simulink model "partieDRL"  (R2024a)
settings: Solver=ode45  StartTime=0.0  StopTime=0.04  RelTol=1e-3  EnableMultiTasking=on
libraries: spsDetailedThyristorLib x16, spsVoltageMeasurementLib x5, spsACVoltageSourceLib x4, spsCurrentMeasurementLib x4, spsDCVoltageSourceLib x4, spsSeriesRLCBranchLib x4, spsDiodeLib x1, spspowerguiLib x1, sps_lib x1
settings Model: Creator=ianyl  LastModifiedBy=ianyl
settings SolverCC: AlgebraicLoopSolver=TrustRegion
settings DataIOCC: LimitDataPoints=on  SaveFormat=Array  ReturnWorkspaceOutputs=off
settings OptimizationCC: LifeSpan=inf
settings DebuggingCC: UnconnectedInputMsg=warning  UnconnectedOutputMsg=warning  UnconnectedLineMsg=warning  SFUnexpectedBacktrackingDiag=warning  SFNoUnconditionalDefaultTransitionDiag=warning  SFExecutionAtInitializationDiag=none  ArithmeticOperatorsInVariantConditions=warning
settings HardwareCC: ProdBitPerPointer=32  ProdBitPerSizeT=32  ProdBitPerPtrDiffT=32  ProdLargestAtomicFloat=None  ProdIntDivRoundTo=Undefined  ProdEndianess=Unspecified  ProdWordSize=32  ProdHWDeviceType=32-bit Generic
settings ModelReferenceCC: PropagateSignalLabelsOutOfModel=off
settings SFSimCC: SimUseLocalCustomCode=off  CustomCodeUndefinedFunction=UseInterfaceOnly
settings RTWCC: RTWUseLocalCustomCode=off  GPUComputeCapability=3.5
settings CodeAppCC: StateflowObjectComments=on
settings GRTTargetCC: TargetLangStandard=C89/C90 (ANSI)
settings ConfigComp: CovMetricSettings=dw  CovSaveCumulativeToWorkspaceVar=on  CovSaveSingleToWorkspaceVar=on  CovExternalEMLEnable=off
settings SimscapeCC: SimscapeNormalizeSystem=off

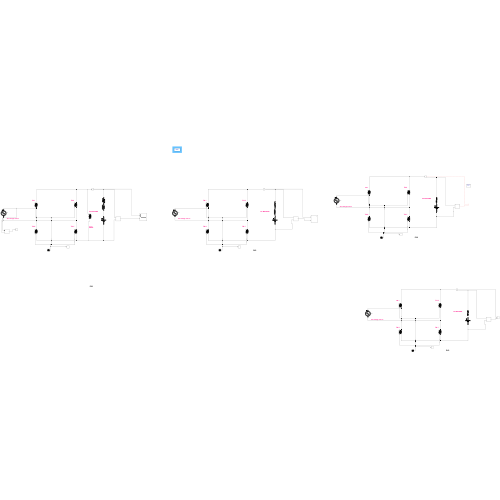
[thumbnail: Simulink's stored preview of the top-level diagram]
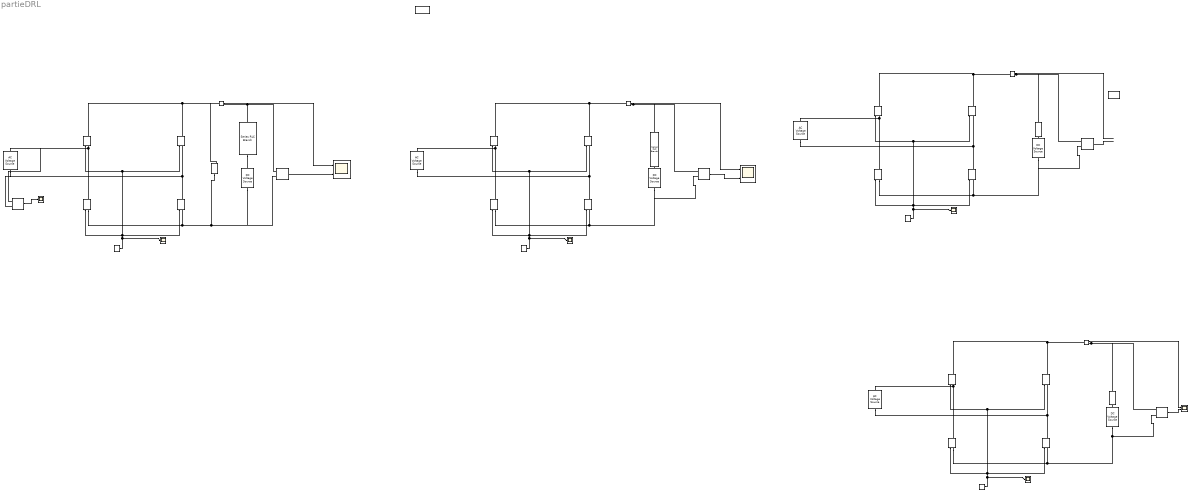
== system partieDRL ==
  note: DRL
  note: PI/3
  note: DC MACHINE
  note: AC voltage source
  note: TH 2'
  note: TH 1'
  note: TH 2
  note: TH 1
  note: PI/2
  note: DC MACHINE
  note: AC voltage source
  note: TH 2'
  note: TH 1'
  note: TH 2
  note: TH 1
  note: PI/2
  note: DC MACHINE
  note: AC voltage source
  note: TH 2'
  note: TH 1'
  note: TH 2
  note: TH 1
  note: PI/2
  note: DC MACHINE
  note: AC voltage source
  note: TH 2'
  note: TH 1'
  note: TH 2
  note: TH 1
  AC : spsACVoltageSourceLib/AC Voltage Source  Amplitude=320.1779  Phase=0  Frequency=50  SampleTime=0  Measurements=None  BusType=swing  Pref=10e3  Qref=0  Qmin=-inf  Qmax=+inf
  AC1 : spsACVoltageSourceLib/AC Voltage Source  Amplitude=320.1779  Phase=0  Frequency=50  SampleTime=0  Measurements=None  BusType=swing  Pref=10e3  Qref=0  Qmin=-inf  Qmax=+inf
  AC2 : spsACVoltageSourceLib/AC Voltage Source  Amplitude=340.4  Phase=0  Frequency=50  SampleTime=0  Measurements=None  BusType=swing  Pref=10e3  Qref=0  Qmin=-inf  Qmax=+inf
  AC3 : spsACVoltageSourceLib/AC Voltage Source  Amplitude=340.4  Phase=0  Frequency=50  SampleTime=0  Measurements=None  BusType=swing  Pref=10e3  Qref=0  Qmin=-inf  Qmax=+inf
  Current Measurement{,1..3} (4 alike) : spsCurrentMeasurementLib/Current Measurement  PhasorSimulation=off  OutputType=Complex  PSBequivalent=0
  DC Voltage Source : spsDCVoltageSourceLib/DC Voltage Source  Amplitude=142.528  Measurements=None
  DC Voltage Source1 : spsDCVoltageSourceLib/DC Voltage Source  Amplitude=92.48  Measurements=None
  DC Voltage Source2 : spsDCVoltageSourceLib/DC Voltage Source  Amplitude=100  Measurements=None
  DC Voltage Source3 : spsDCVoltageSourceLib/DC Voltage Source  Amplitude=100  Measurements=None
  Detailed Thyristor{,1..15} (16 alike) : spsDetailedThyristorLib/Detailed Thyristor  Ron=0.001  Lon=1e-3  Vf=0.8  IL=0.1  Tq=100e-6  IC=0  Rs=500  Cs=250e-9  Measurements=on
      settings: LibrarySourceBlock=sps_lib/Power Electronics/Detailed Thyristor
  Diode : spsDiodeLib/Diode  Ron=0.001  Lon=0  Vf=0.8  IC=0  UseSnubber=off  Rs=500  Cs=250e-9  Measurements=on
  Pulse Generator : DiscretePulseGenerator  PulseType=Time based  Amplitude=5  Period=0.01  PulseWidth=30  PhaseDelay=3.333333*10^(-3)
  Pulse Generator2 : DiscretePulseGenerator  PulseType=Time based  Amplitude=5  Period=0.01  PulseWidth=30  PhaseDelay=5*10^(-3)
  Pulse Generator3 : DiscretePulseGenerator  PulseType=Time based  Amplitude=5  Period=0.01  PulseWidth=30  PhaseDelay=5*10^(-3)
  Pulse Generator4 : DiscretePulseGenerator  PulseType=Time based  Amplitude=5  Period=0.01  PulseWidth=30  PhaseDelay=5*10^(-3)
  Scope : Scope  NumInputPorts=2
  Scope{1..2,4..6} (5 alike) : Scope
  Scope3 : Scope  NumInputPorts=2
  Scope7 : Scope  NumInputPorts=2
  Series RLC Branch : spsSeriesRLCBranchLib/Series RLC Branch  LConnTagsString=__new0  RConnTagsString=__new0  BranchType=RL  Resistance=2.33  Inductance=0.055  SetiL0=off  InitialCurrent=0  Capacitance=1e-6  Setx0=off  InitialVoltage=0  Measurements=None
  Series RLC Branch1 : spsSeriesRLCBranchLib/Series RLC Branch  LConnTagsString=__new0  RConnTagsString=__new0  BranchType=RL  Resistance=2.33  Inductance=0.286  SetiL0=off  InitialCurrent=0  Capacitance=1e-6  Setx0=off  InitialVoltage=0  Measurements=None
  Series RLC Branch2 : spsSeriesRLCBranchLib/Series RLC Branch  LConnTagsString=__new0  RConnTagsString=__new0  BranchType=RL  Resistance=2.33  Inductance=1e-3  SetiL0=off  InitialCurrent=0  Capacitance=1e-6  Setx0=off  InitialVoltage=0  Measurements=None
  Series RLC Branch3 : spsSeriesRLCBranchLib/Series RLC Branch  LConnTagsString=__new0  RConnTagsString=__new0  BranchType=RL  Resistance=2.33  Inductance=288e-3  SetiL0=off  InitialCurrent=0  Capacitance=1e-6  Setx0=off  InitialVoltage=0  Measurements=None
  Voltage Measurement{,1..4} (5 alike) : spsVoltageMeasurementLib/Voltage Measurement  PhasorSimulation=off  OutputType=Complex  PSBequivalent=0
  powergui : spspowerguiLib/powergui  Priority=1  SimulationMode=Discrete  SampleTime=50e-6  frequency=60  Iterations=50  frequencyindice=0  Pbase=100e6  ErrMax=1e-4  UnitsV=kV  UnitsW=MW  buscounter=0  FunctionMessages=off  echomessages=off  EnableUseOfTLC=off  CurrentSourceSwitches=off  DisableSnubberDevices=off  DisableRonSwitches=off  DisableVfSwitches=off  DisplayEquations=off  AutomaticDiscreteSolvers=off  SolverType=Tustin/Backward Euler (TBE)  Interpol=off  ExternalGateDelay=off  methode=off  Ts=100  x0status=blocks  SPID=off  SwTol=0  HookPort=off  NonlinearTolerance=1e-4  nMaxIteration=100  ContinueOnMaxIteration=off  RestoreLinks=warning  ResistiveCurrentMeasurement=off  Frange=[0:2:500]  Ylog=off  Xlog=on  ShowGrid=off  save=off  variable=ZData  structure=0  ZoomFFT=off  StartTime=0.0  cycles=1  DisplayStyle=1  fundamental=60  FreqAxis=off  MaxFrequency=1000  frequencyindicesteady=1  RmsSteady=1  display=off
  powergui1 : sps_lib/powergui  Priority=1  SimulationMode=Discrete  SampleTime=50e-6  frequency=60  Iterations=50  frequencyindice=50  Pbase=100e6  ErrMax=1e-4  UnitsV=kV  UnitsW=MW  buscounter=0  FunctionMessages=off  echomessages=off  EnableUseOfTLC=off  CurrentSourceSwitches=off  DisableSnubberDevices=off  DisableRonSwitches=off  DisableVfSwitches=off  DisplayEquations=off  AutomaticDiscreteSolvers=off  SolverType=Tustin/Backward Euler (TBE)  Interpol=off  ExternalGateDelay=off  methode=off  Ts=100  x0status=blocks  SPID=on  SwTol=0  HookPort=off  NonlinearTolerance=1e-4  nMaxIteration=100  ContinueOnMaxIteration=off  RestoreLinks=warning  ResistiveCurrentMeasurement=off  Frange=[0:2:500]  Ylog=off  Xlog=on  ShowGrid=off  save=off  variable=ZData  structure=0  ZoomFFT=off  StartTime=0.0  cycles=1  DisplayStyle=1  fundamental=60  FreqAxis=off  MaxFrequency=1000  frequencyindicesteady=1  RmsSteady=1  display=off
  wires:
  Voltage Measurement/1 -> Scope/2
  Current Measurement/1 -> Scope/1
  Pulse Generator/1 -> Scope1/1, Detailed Thyristor3/1, Detailed Thyristor1/1, Detailed Thyristor/1, Detailed Thyristor2/1
  Voltage Measurement1/1 -> Scope3/2
  Current Measurement1/1 -> Scope3/1
  Pulse Generator2/1 -> Scope4/1, Detailed Thyristor7/1, Detailed Thyristor5/1, Detailed Thyristor4/1, Detailed Thyristor6/1
  Voltage Measurement2/1 -> ?
  Current Measurement2/1 -> ?
  Pulse Generator3/1 -> Scope5/1, Detailed Thyristor11/1, Detailed Thyristor9/1, Detailed Thyristor8/1, Detailed Thyristor10/1
  Voltage Measurement3/1 -> Scope7/2
  Current Measurement3/1 -> Scope7/1
  Pulse Generator4/1 -> Scope6/1, Detailed Thyristor13/1, Detailed Thyristor15/1, Detailed Thyristor14/1, Detailed Thyristor12/1
  Voltage Measurement4/1 -> Scope2/1
  connections:
  Detailed Thyristor2/RConn1 -- Voltage Measurement4/LConn1 -- AC/RConn1 -- Detailed Thyristor/LConn1
  Detailed Thyristor/RConn1 -- Diode/RConn1 -- Current Measurement/LConn1 -- Detailed Thyristor1/RConn1
  Detailed Thyristor3/RConn1 -- Voltage Measurement4/LConn2 -- AC/LConn1 -- Detailed Thyristor1/LConn1
  Detailed Thyristor2/LConn1 -- Diode/LConn1 -- DC Voltage Source/LConn1 -- Voltage Measurement/LConn2 -- Detailed Thyristor3/LConn1
  Series RLC Branch/LConn1 -- Voltage Measurement/LConn1 -- Current Measurement/RConn1
  Series RLC Branch/RConn1 -- DC Voltage Source/RConn1
  Detailed Thyristor6/RConn1 -- AC1/RConn1 -- Detailed Thyristor4/LConn1
  Detailed Thyristor4/RConn1 -- Current Measurement1/LConn1 -- Detailed Thyristor5/RConn1
  Detailed Thyristor7/RConn1 -- AC1/LConn1 -- Detailed Thyristor5/LConn1
  Detailed Thyristor6/LConn1 -- DC Voltage Source1/LConn1 -- Voltage Measurement1/LConn2 -- Detailed Thyristor7/LConn1
  Current Measurement1/RConn1 -- Series RLC Branch1/LConn1 -- Voltage Measurement1/LConn1
  Series RLC Branch1/RConn1 -- DC Voltage Source1/RConn1
  Detailed Thyristor10/RConn1 -- AC2/RConn1 -- Detailed Thyristor8/LConn1
  Detailed Thyristor8/RConn1 -- Current Measurement2/LConn1 -- Detailed Thyristor9/RConn1
  Detailed Thyristor11/RConn1 -- AC2/LConn1 -- Detailed Thyristor9/LConn1
  Detailed Thyristor10/LConn1 -- Detailed Thyristor11/LConn1 -- DC Voltage Source2/LConn1 -- Voltage Measurement2/LConn2
  Current Measurement2/RConn1 -- Series RLC Branch2/LConn1 -- Voltage Measurement2/LConn1
  Series RLC Branch2/RConn1 -- DC Voltage Source2/RConn1
  Detailed Thyristor12/RConn1 -- AC3/RConn1 -- Detailed Thyristor14/LConn1
  Detailed Thyristor14/RConn1 -- Current Measurement3/LConn1 -- Detailed Thyristor15/RConn1
  Detailed Thyristor13/RConn1 -- AC3/LConn1 -- Detailed Thyristor15/LConn1
  Voltage Measurement3/LConn2 -- DC Voltage Source3/LConn1 -- Detailed Thyristor13/LConn1 -- Detailed Thyristor12/LConn1
  Current Measurement3/RConn1 -- Series RLC Branch3/LConn1 -- Voltage Measurement3/LConn1
  Series RLC Branch3/RConn1 -- DC Voltage Source3/RConn1
